simulink model "bloquesT3"  (R2022b)
settings: Solver=VariableStepAuto  StartTime=0.0  StopTime=10  RelTol=1e-3
model workspace (MAT data in the model file):
  b1 = 1000
  m1 = 290
values from neighbouring files (symbols this model uses):
  k1 = 16182    [DobleP1.m]    (also in Tarea3.m)
  k2 = 19000    [DobleP1.m]    (also in Tarea3.m)
  m2 = 59    [DobleP1.m]    (also in Tarea3.m)
settings Model: Creator=Sofia.Landa  LastModifiedBy=Sofia.Landa

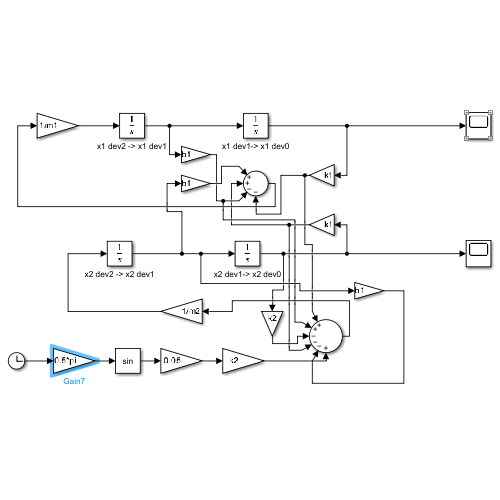
[thumbnail: Simulink's stored preview of the top-level diagram]
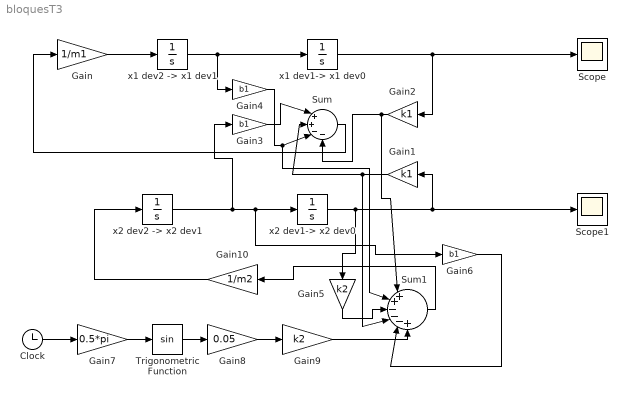
== system bloquesT3 ==
  Clock : Clock
  Gain : Gain  Gain=1/m1
  Gain1 : Gain  Gain=k1
  Gain10 : Gain  Gain=1/m2
  Gain2 : Gain  Gain=k1
  Gain3 : Gain  Gain=b1
  Gain4 : Gain  Gain=b1
  Gain5 : Gain  Gain=k2
  Gain6 : Gain  Gain=b1
  Gain7 : Gain  Gain=0.5*pi
  Gain8 : Gain  Gain=0.05
  Gain9 : Gain  Gain=k2
  Scope : Scope
  Scope1 : Scope
  Sum : Sum  Inputs=|++--
  Sum1 : Sum  Inputs=|++---+
  Trigonometric Function : Trigonometry
  x1 dev1-> x1 dev0 : Integrator
  "x1 dev2 -> x1 dev1" : Integrator
  x2 dev1-> x2 dev0 : Integrator
  "x2 dev2 -> x2 dev1" : Integrator
  wires:
  "x1 dev2 -> x1 dev1"/1 -> Gain4/1, x1 dev1-> x1 dev0/1
  "x2 dev2 -> x2 dev1"/1 -> Gain3/1, Gain6/1, x2 dev1-> x2 dev0/1
  Gain/1 -> "x1 dev2 -> x1 dev1"/1
  Gain2/1 -> Sum/4, Sum1/1
  x2 dev1-> x2 dev0/1 -> Gain5/1, Scope1/1, Gain1/1
  x1 dev1-> x1 dev0/1 -> Gain2/1, Scope/1
  Gain1/1 -> Sum/2, Sum1/4
  Gain3/1 -> Sum/1
  Gain4/1 -> Sum1/2, Sum/3
  Gain5/1 -> Sum1/3
  Gain6/1 -> Sum1/5
  Sum/1 -> Gain/1
  Clock/1 -> Gain7/1
  Gain7/1 -> Trigonometric Function/1
  Trigonometric Function/1 -> Gain8/1
  Gain8/1 -> Gain9/1
  Gain9/1 -> Sum1/6
  Sum1/1 -> Gain10/1
  Gain10/1 -> "x2 dev2 -> x2 dev1"/1
